simulink model "BMSRC2"  (R2026a)
settings: Solver=ode15s  StopTime=100
libraries: simulink x2, SignalEditorBlockLib x1
settings Model: Creator=manoj  LastModifiedBy=manoj

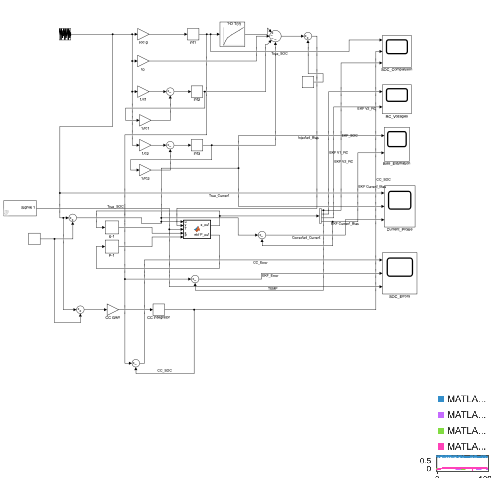
[thumbnail: Simulink's stored preview of the top-level diagram]
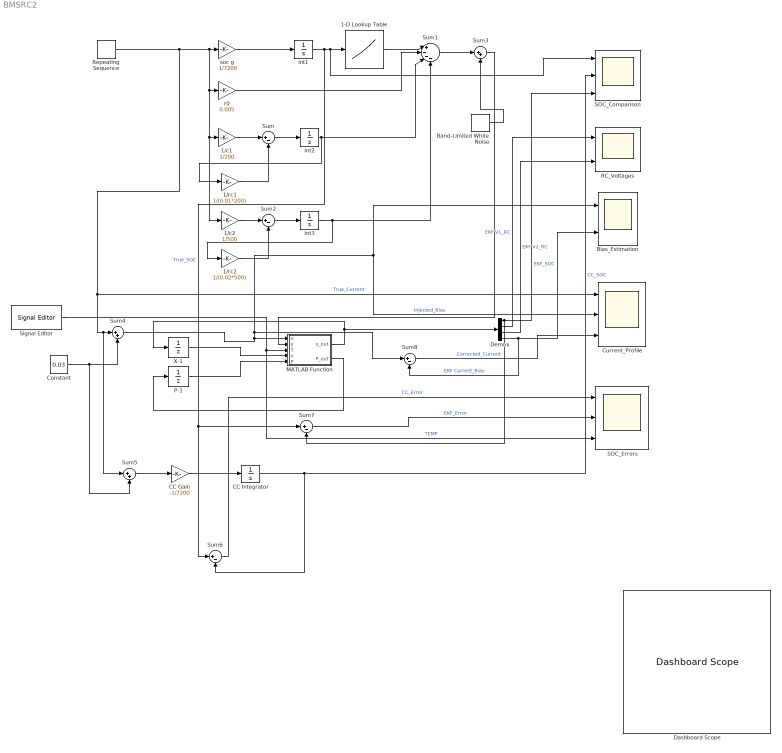
== system BMSRC2 ==
  1-D Lookup Table : Lookup_n-D  NumberOfTableDimensions=1  BreakpointsForDimension1=[0 0.1 0.2 0.4 0.6 0.8 1]  Table=[3.0 3.3 3.5 3.7 3.85 4.0 4.2]  InternalRulePriority=Speed  RndMeth=Simplest
  1/c1 : Gain  Gain=1/200
  1/c2 : Gain  Gain=1/500
  1/rc1 : Gain  Gain=1/(0.01*200)
  1/rc2 : Gain  Gain=1/(0.02*500)
  Band-Limited White Noise : simulink/Sources/Band-Limited White Noise  Cov=1e-6  Ts=0.01  seed=[23341]
  Bias_Estimation : Scope  NumInputPorts=2
      settings: ActiveDisplayYMinimum=-2.7199999999999998  ActiveDisplayYMaximum=4.78  DataLoggingVariableName=ScopeData4
  CC Gain : Gain  Gain=-1/7200
  CC Integrator : Integrator  InitialCondition=0.8
  Constant : Constant  Value=0.03
  Current_Profile : Scope  NumInputPorts=3
      settings: ActiveDisplayYMinimum=-2.760556613471234  ActiveDisplayYMaximum=4.7845062903856928  DataLoggingVariableName=ScopeData5
  Dashboard Scope : DashboardScope  FontColor=[0.0, 0.0, 0.0]
  Demux : Demux
  Int2 : Integrator
  Int3 : Integrator
  MATLAB Function : MATLAB Function  TreatAsAtomicUnit=on
  P-1 : UnitDelay  InitialCondition=eye(4)*1e-3  SampleTime=-1
  RC_Voltages : Scope  NumInputPorts=2
      settings: ActiveDisplayYMinimum=-0.023317260712214904  ActiveDisplayYMaximum=0.05471790189091412  DataLoggingVariableName=ScopeData3
  Repeating Sequence : simulink/Sources/Repeating Sequence  rep_seq_t=[0 10 20 30 40 50 60 70 80 90 100]  rep_seq_y=[2 4 1 3 -2 4 0.5 3 -1 2 0]
  SOC_Comparison : Scope  NumInputPorts=3
      settings: ActiveDisplayYMinimum=0.75055585873226571  ActiveDisplayYMaximum=0.82828775731892534  DataLoggingVariableName=ScopeData6
  SOC_Errors : Scope  NumInputPorts=3
      settings: ActiveDisplayYMinimum=-5.2083333333369217E-5  ActiveDisplayYMaximum=0.00046875000000032307
  Signal Editor : SignalEditorBlockLib/Signal Editor  FileName=untitled.mat  ActiveScenario=Scenario  ActiveSignal=Signal 1  IsBus=off  OutputBusObjectStr=Bus: BusObject  SampleTime=0  ZeroCross=off  OutputAfterFinalValue=Setting to zero  Unit=inherit  PreserveSignalName=on  ApplySigPropsToAllScenarios=on  ApplySigPropsToAllSignals=off  SignalPropertySource=Dialog parameters
  Sum{,2,6..8} (5 alike) : Sum  Inputs=|+-
  Sum1 : Sum  Inputs=|+---
  Sum3 : Sum  Inputs=|++
  Sum4 : Sum  Inputs=|++
  Sum5 : Sum  Inputs=|++
  X-1 : UnitDelay  InitialCondition=[0.8; 0; 0; 0]  SampleTime=-1
  int1 : Integrator  InitialCondition=0.8  LimitOutput=on  UpperSaturationLimit=1  LowerSaturationLimit=0
  "r0 " : Gain  Gain=0.005
  soc g : Gain  Gain=-1/7200
  wires:
  Sum2/1 -> Int3/1
  soc g/1 -> int1/1
  Sum1/1 -> Sum3/1
  1-D Lookup Table/1 -> Sum1/1
  Int2/1 -> 1/rc1/1, Sum1/3
  "r0 "/1 -> Sum1/2
  X-1/1 -> MATLAB Function/4(x)
  1/c1/1 -> Sum/1
  int1/1 -> Sum7/1, Sum6/1, SOC_Comparison/1, 1-D Lookup Table/1  "True_SOC"
  1/rc2/1 -> Sum2/2
  Band-Limited White Noise/1 -> Sum3/2
  Sum/1 -> Int2/1
  Int3/1 -> 1/rc2/1, Sum1/4
  MATLAB Function/2(P_out) -> P-1/1
  1/c2/1 -> Sum2/1
  1/rc1/1 -> Sum/2
  Sum3/1 -> MATLAB Function/2(y)
  P-1/1 -> MATLAB Function/5(P)
  Constant/1 -> Sum5/2, Sum4/2
  Sum4/1 -> Sum8/1, Bias_Estimation/1, Current_Profile/2, MATLAB Function/1(u)  "Injected_Bias"
  CC Gain/1 -> CC Integrator/1
  Sum5/1 -> CC Gain/1
  MATLAB Function/1(x_out) -> X-1/1, Demux/1
  Signal Editor/1 -> SOC_Errors/3, MATLAB Function/3(T)  "TEMP"
  Demux/4 -> Sum8/2, Bias_Estimation/2  "EKF Current_Bias"
  Demux/3 -> RC_Voltages/2  "EKF V2_RC"
  Demux/2 -> RC_Voltages/1  "EKF V1_RC"
  Demux/1 -> Sum7/2, SOC_Comparison/3  "EKF_SOC"
  CC Integrator/1 -> SOC_Comparison/2, Sum6/2  "CC_SOC"
  Repeating Sequence/1 -> Current_Profile/1, Sum5/1, Sum4/1, 1/c2/1, 1/c1/1, "r0 "/1, soc g/1  "True_Current"
  Sum6/1 -> SOC_Errors/1  "CC_Error"
  Sum7/1 -> SOC_Errors/2  "EKF_Error"
  Sum8/1 -> Current_Profile/3  "Corrected_Current"

== matlab function BMSRC2/MATLAB Function ==
  data: u input; x_out output; y input; T input; x input; P input; P_out output
function [x_out, P_out] = ekf(u, y, T, x, P)

Ts = 0.01;

% ---- Parameters ----
R0_ref = 0.005;
R1_ref = 0.01;
R2_ref = 0.02;

alpha0 = 0.03;
alpha1 = 0.05;
alpha2 = 0.05;

R0 = R0_ref*(1 + alpha0*(25 - T));
R1 = R1_ref*(1 + alpha1*(25 - T));
R2 = R2_ref*(1 + alpha2*(25 - T));

Qb = 7200;

C1 = 200;
C2 = 500;

a1 = exp(-Ts/(R1*C1));
a2 = exp(-Ts/(R2*C2));

% ---- States ----
SOC = x(1);
V1  = x(2);
V2  = x(3);
bias = x(4);   % NEW

I_meas = u;

% ---- Prediction ----
SOC_pred = SOC - Ts/Qb * (I_meas - bias);   % corrected current
V1_pred  = a1*V1 + R1*(1-a1)*(I_meas - bias);
V2_pred  = a2*V2 + R2*(1-a2)*(I_meas - bias);

bias_pred = bias;  % bias assumed slowly varying

x_pred = [SOC_pred; V1_pred; V2_pred; bias_pred];

% ---- OCV lookup ----
soc_bp = [0 0.1 0.2 0.4 0.6 0.8 1];
ocv_bp = [3.0 3.3 3.5 3.7 3.85 4.0 4.2];

OCV = interp1(soc_bp, ocv_bp, SOC_pred, 'linear', 'extrap');

% ---- Output prediction ----
y_pred = OCV - R0*(I_meas - bias) - V1_pred - V2_pred;

% ---- dOCV/dSOC ----
dSOC = 1e-4;
OCV_p = interp1(soc_bp, ocv_bp, SOC_pred + dSOC,'linear','extrap');
OCV_m = interp1(soc_bp, ocv_bp, SOC_pred - dSOC,'linear','extrap');

dOCV = (OCV_p - OCV_m)/(2*dSOC);

% ---- Jacobians ----
F = [1 0 0 Ts/Qb;
     0 a1 0 -R1*(1-a1);
     0 0 a2 -R2*(1-a2);
     0 0 0 1];

H = [dOCV  -1  -1   R0];

% ---- Noise tuning ----
Qk = diag([1e-6, 5e-7, 5e-7, 5e-5]);   % bias gets higher uncertainty
Rk = 5e-5;

% ---- Covariance ----
P_pred = F*P*F' + Qk;

% ---- Kalman Gain ----
K = P_pred*H'/(H*P_pred*H' + Rk);

% ---- Update ----
x_out = x_pred + K*(y - y_pred);

P_out = (eye(4) - K*H)*P_pred;
x_out(4) = max(min(x_out(4),0.1),-0.1);

end
